simulink model "Exemplu1_sim"  (R2024b)
settings: Solver=VariableStepAuto  StartTime=0.0  StopTime=20.0  RelTol=1e-3
values from neighbouring files (symbols this model uses):
  a = 1    [Exercitii_lab.m]
  c = 1    [Exercitii_lab.m]
  d = 2    [Exercitii_lab.m]
  x1 = 1.5    [Exemplu1.m]
  y1 = 2    [Exemplu1.m]
  y2 = 1    [Exemplu1.m]
settings Model: Creator=akopo  LastModifiedBy=akopo

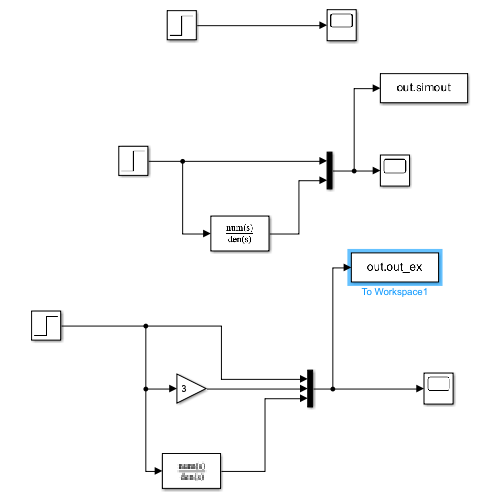
[thumbnail: Simulink's stored preview of the top-level diagram]
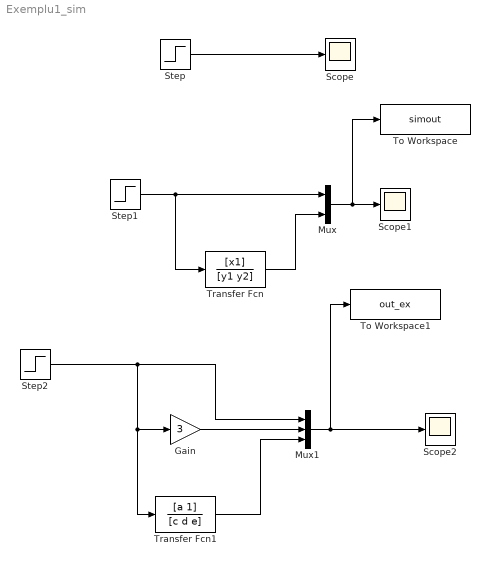
== system Exemplu1_sim ==
  Gain : Gain  Gain=3
  Mux : Mux  Inputs=2
  Mux1 : Mux  Inputs=3
  Scope : Scope
  Scope1 : Scope
  Scope2 : Scope
  Step : Step  SampleTime=0
  Step1 : Step  SampleTime=0
  Step2 : Step  Time=5  Before=2  After=4  SampleTime=0
  To Workspace : ToWorkspace  VariableName=simout  SaveFormat=Timeseries  SampleTime=-1
  To Workspace1 : ToWorkspace  VariableName=out_ex  SaveFormat=Timeseries  SampleTime=-1
  Transfer Fcn : TransferFcn  Numerator=[x1]  Denominator=[y1 y2]
  Transfer Fcn1 : TransferFcn  Numerator=[a 1]  Denominator=[c d e]
  wires:
  Step/1 -> Scope/1
  Step1/1 -> Transfer Fcn/1, Mux/1
  Mux/1 -> To Workspace/1, Scope1/1
  Transfer Fcn/1 -> Mux/2
  Mux1/1 -> Scope2/1, To Workspace1/1
  Step2/1 -> Gain/1, Transfer Fcn1/1, Mux1/1
  Gain/1 -> Mux1/2
  Transfer Fcn1/1 -> Mux1/3
